simulink model "Prob02"  (R2020a)
settings: Solver=VariableStepAuto  StartTime=0.0  StopTime=10.0  RelTol=1e-3
model workspace (MAT data in the model file):
  Ie = Simulink.Parameter
  Ie.Value = 1
  Ie.DataType = 'auto'
  Ie.Dimensions = [1 1]
  Iv = Simulink.Parameter
  Iv.Value = 1
  Iv.DataType = 'auto'
  Iv.Dimensions = [1 1]
  be = Simulink.Parameter
  be.Value = 1
  be.DataType = 'auto'
  be.Dimensions = [1 1]
  bv = Simulink.Parameter
  bv.Value = 1
  bv.DataType = 'auto'
  bv.Dimensions = [1 1]
settings Model: Creator=Shivam  LastModifiedBy=Shivam

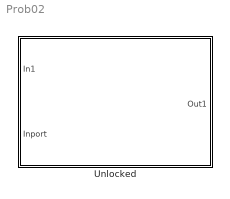
== system Prob02 ==
  Unlocked : Subsystem

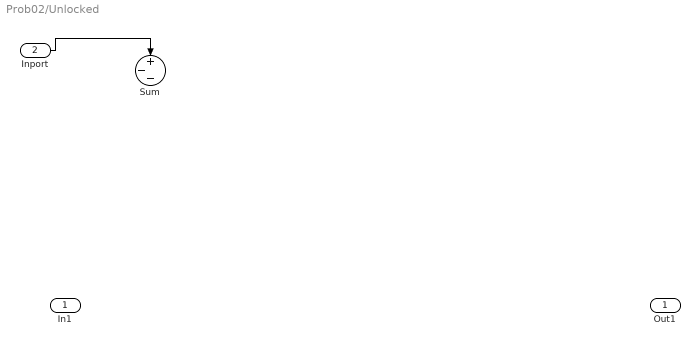
== system Prob02/Unlocked ==
  In1 : Inport
  Inport : Inport  Port=2
  Sum : Sum  Inputs=+--
  Out1 : Outport
  wires:
  Inport/1 -> Sum/1
